simulink model "SallenKey"  (R2015a)
settings: Solver=ode45  StartTime=0.0  StopTime=10  RelTol=1e-3
settings Model: Creator=Abel  LastModifiedBy=abeel

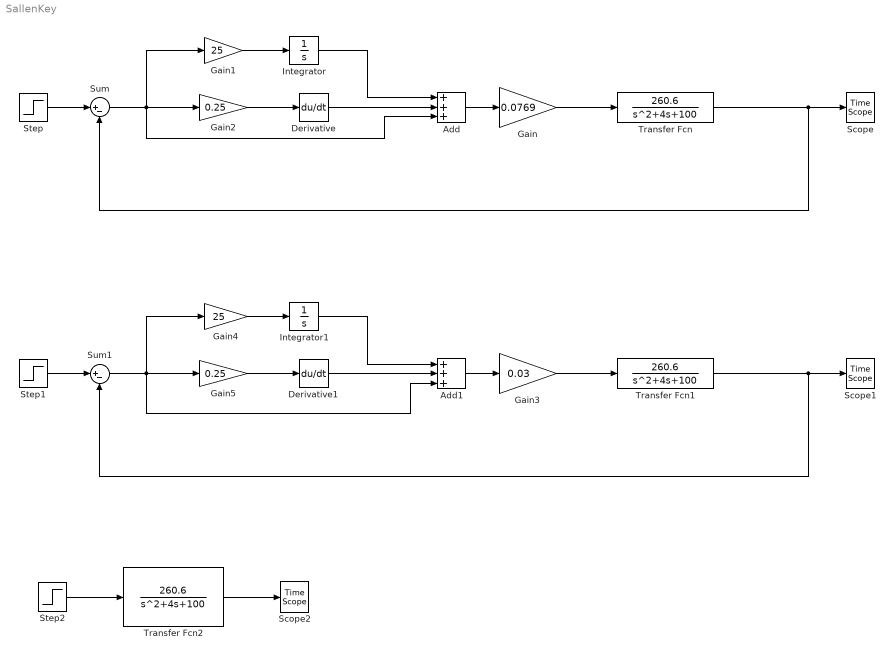
== system SallenKey ==
  Add : Sum  Inputs=+++
  Add1 : Sum  Inputs=+++
  Derivative : Derivative
  Derivative1 : Derivative
  Gain : Gain  Gain=0.0769
  Gain1 : Gain  Gain=25
  Gain2 : Gain  Gain=0.25
  Gain3 : Gain  Gain=0.03
  Gain4 : Gain  Gain=25
  Gain5 : Gain  Gain=0.25
  Integrator : Integrator
  Integrator1 : Integrator
  Scope : TimeScope
  Scope1 : TimeScope
  Scope2 : TimeScope
  Step : Step  Time=0  SampleTime=0
  Step1 : Step  Time=0  SampleTime=0
  Step2 : Step  Time=0  SampleTime=0
  Sum : Sum  Inputs=|+-
  Sum1 : Sum  Inputs=|+-
  Transfer Fcn : TransferFcn  Numerator=[260.6]  Denominator=[1 4 100]
  Transfer Fcn1 : TransferFcn  Numerator=[260.6]  Denominator=[1 4 100]
  Transfer Fcn2 : TransferFcn  Numerator=[260.6]  Denominator=[1 4 100]
  wires:
  Transfer Fcn/1 -> Sum/2, Scope/1
  Step/1 -> Sum/1
  Gain1/1 -> Integrator/1
  Integrator/1 -> Add/1
  Gain2/1 -> Derivative/1
  Derivative/1 -> Add/2
  Sum/1 -> Gain1/1, Gain2/1, Add/3
  Add/1 -> Gain/1
  Gain/1 -> Transfer Fcn/1
  Transfer Fcn1/1 -> Sum1/2, Scope1/1
  Step1/1 -> Sum1/1
  Gain4/1 -> Integrator1/1
  Integrator1/1 -> Add1/1
  Gain5/1 -> Derivative1/1
  Derivative1/1 -> Add1/2
  Add1/1 -> Gain3/1
  Gain3/1 -> Transfer Fcn1/1
  Step2/1 -> Transfer Fcn2/1
  Transfer Fcn2/1 -> Scope2/1
  Sum1/1 -> Add1/3, Gain4/1, Gain5/1
